simulink model "pendulo"  (Simulink 10.1)
settings: Solver=VariableStepAuto  StartTime=0.0  StopTime=stop_time  RelTol=1e-6
values from neighbouring files (symbols this model uses):
  g = 9.8    [caotico.m]    (also in lab1.m; teste_pendulo.m)
  l = 0.5    [caotico.m]    (also in lab1.m; natureza.m = legend(plotHandles, plotLabels, 'Location', 'best'); teste_pendulo.m)
  m = 1    [caotico.m]    (also in lab1.m; teste_pendulo.m)
  p1_0 = (1/6)*m*(l^2)*(8*d_th1_0+3*d_th2_0*cos(theta1_0-theta2_0))    [caotico.m]    (also in lab1.m; teste_pendulo.m = 0)
  p2_0 = (1/6)*m*(l^2)*(2*d_th2_0+3*d_th1_0*cos(theta1_0-theta2_0))    [caotico.m]    (also in lab1.m; teste_pendulo.m = 0)
  theta1_0 = small_th1(i)    [caotico.m]    (also in lab1.m; teste_pendulo.m = 3)
  theta2_0 = small_th2(i)    [caotico.m]    (also in lab1.m; teste_pendulo.m = -2.5)
settings Model: Creator=Daniel  LastModifiedBy=Daniel
settings DataIOCC: SaveFormat=Dataset  ReturnWorkspaceOutputs=on
settings OptimizationCC: LifeSpan=auto
settings DebuggingCC: UnderspecifiedInitializationDetection=Simplified  MergeDetectMultiDrivingBlocksExec=error  SFUnexpectedBacktrackingDiag=error  SFNoUnconditionalDefaultTransitionDiag=error  SFExecutionAtInitializationDiag=warning  ArithmeticOperatorsInVariantConditions=error
settings HardwareCC: ProdBitPerPointer=64  ProdBitPerSizeT=64  ProdBitPerPtrDiffT=64  ProdLargestAtomicFloat=Float  ProdIntDivRoundTo=Zero  ProdEndianess=LittleEndian  ProdWordSize=64  ProdHWDeviceType=Intel->x86-64 (Windows64)
settings ModelReferenceCC: PropagateSignalLabelsOutOfModel=on
settings SFSimCC: SimUseLocalCustomCode=on  CustomCodeUndefinedFunction=FilterOut
settings RTWCC: RTWUseLocalCustomCode=on
settings CodeAppCC: StateflowObjectComments=off
settings GRTTargetCC: TargetLangStandard=C99 (ISO)  CombineOutputUpdateFcns=on  GRTInterface=off
settings ConfigComp: CovMetricSettings=dwe  CovHtmlReporting=off  CovSaveCumulativeToWorkspaceVar=off  CovSaveSingleToWorkspaceVar=off  CovExternalEMLEnable=on

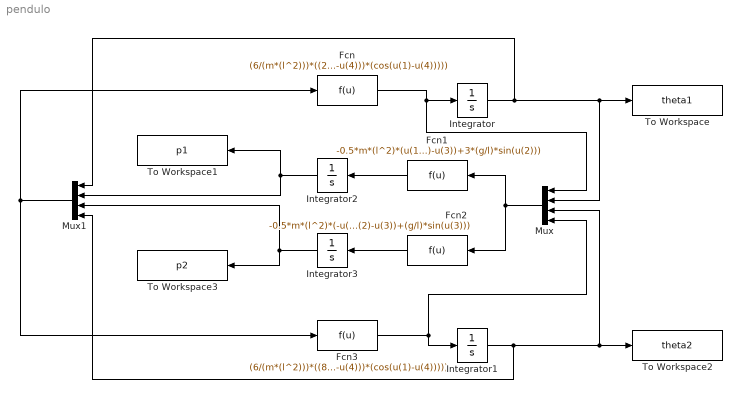
== system pendulo ==
  Fcn : Fcn  Expr=(6/(m*(l^2)))*((2*u(2)-3*cos(u(1)-u(4))*u(3))/(16-9*(cos(u(1)-u(4)))*(cos(u(1)-u(4)))))
  Fcn1 : Fcn  Expr=-0.5*m*(l^2)*(u(1)*u(4)*sin(u(2)-u(3))+3*(g/l)*sin(u(2)))
  Fcn2 : Fcn  Expr=-0.5*m*(l^2)*(-u(1)*u(4)*sin(u(2)-u(3))+(g/l)*sin(u(3)))
  Fcn3 : Fcn  Expr=(6/(m*(l^2)))*((8*u(3)-3*cos(u(1)-u(4))*u(2))/(16-9*(cos(u(1)-u(4)))*(cos(u(1)-u(4)))))
  Integrator : Integrator  InitialCondition=theta1_0
  Integrator1 : Integrator  InitialCondition=theta2_0
  Integrator2 : Integrator  InitialCondition=p1_0
  Integrator3 : Integrator  InitialCondition=p2_0
  Mux : Mux
  Mux1 : Mux
  To Workspace : ToWorkspace  VariableName=theta1  SampleTime=-1
  To Workspace1 : ToWorkspace  VariableName=p1  SampleTime=-1
  To Workspace2 : ToWorkspace  VariableName=theta2  SampleTime=-1
  To Workspace3 : ToWorkspace  VariableName=p2  SampleTime=-1
  wires:
  Mux/1 -> Fcn2/1, Fcn1/1
  Fcn1/1 -> Integrator2/1
  Fcn2/1 -> Integrator3/1
  Integrator2/1 -> To Workspace1/1, Mux1/2
  Integrator3/1 -> To Workspace3/1, Mux1/3
  Integrator/1 -> Mux1/1, To Workspace/1, Mux/2
  Fcn/1 -> Integrator/1, Mux/1
  Integrator1/1 -> Mux/3, To Workspace2/1, Mux1/4
  Fcn3/1 -> Integrator1/1, Mux/4
  Mux1/1 -> Fcn3/1, Fcn/1
